simulink model "Eingangs_Ausgangs_Linearisierung_U1_2024b"  (R2024b)
settings: Solver=VariableStepAuto  StartTime=0.0  StopTime=10  MaxStep=1e-3
InitFcn:
  | clear all;
  | 
  | R = 1e+3;
  | L = 100e-3;
  | C1 = 100e-9;
  | C2 = 1e-6;
  | 
  | k  = 1.380649e-23;
  | e  = 1.602176634e-19;
  | T  = 25 + 273.15;
  | UT = k*T/e;
  | IS = 10e-9;
  | 
  | U0 = 12;
  | I0 = 10e-3;
  | 
  | syms U1 U2 IL
  | x = [U1, U2, IL];
  | 
  | %Zerlegung für Linearisierung
  | f = [-IS*exp(-U2/UT)/C1 + IL/C1;
  |      IL/C2;
  |      -U1/L - U2/L - R*IL/L];
  | 
  | g = [0, 0;
  |      0, -1/C2;
  |      1/L, 0];
  | 
  | h = U1;
  | 
  | %Lie-Ableitungen
  | Lf = h;
  | Lf_h = Lf;
  | 
  | Lf_r_init = sym(zeros(10,1));
  | Lf_r_init(1) = Lf_h;
  | 
  | r = 0;
  | 
  | 
  | while true
  | 
  |     LgLf = jacobian(Lf, x) * g;
  | 
  |     if (LgLf(1) ~= 0 || LgLf(2) ~= 0)
  |         Lf = jacobian(Lf, x) * f;
  |         Lf_h = Lf;
  |         break;
  |     end
  | 
  |     Lf = jacobian(Lf, x) * f;
  |     Lf_h = Lf;
  |     Lf_r_init(r+2) = Lf_h;
  |     r = r + 1;
  | 
  | end
  | 
  | r = r + 1
  | 
  | if r == 1
  | 
  |     Lf_r = zeros(1,1);
  |     Lf_r = Lf_r_init(1);
  | 
  |     % Pol für Regelung
  |     p = -3;
  | 
  | end
  | 
  | if r == 2
  | 
  |     Lf_r = zeros(2,1);
  |     Lf_r = Lf_r_init(1:2);
  | 
  |     % Pole für Regelung
  |     p = [-2-2*i, -2+2*i];
  | 
  | end
  | 
  | phi = Lf_r
  | 
  | alpha = LgLf;
  | alpha_pinv = pinv(alpha)
  | 
  | beta = Lf_h
  | 
  | A = zeros(r);
  | for i=1:r
  |     for j=1:r
  |         if j == i+1
  |             A(i,j) = 1;
  |         end
  |     end
  | end
  | 
  | A
  | 
  | B = zeros(r,1);
  | B(r) = 1
  | 
  | C = zeros(1,r);
  | C(1) = 1
  | 
  | p
  | 
  | G = place(A, B, p)
settings Model: Creator=richa  LastModifiedBy=richa
settings ConfigComp: CovBoundaryAbsTol=1.0e-5

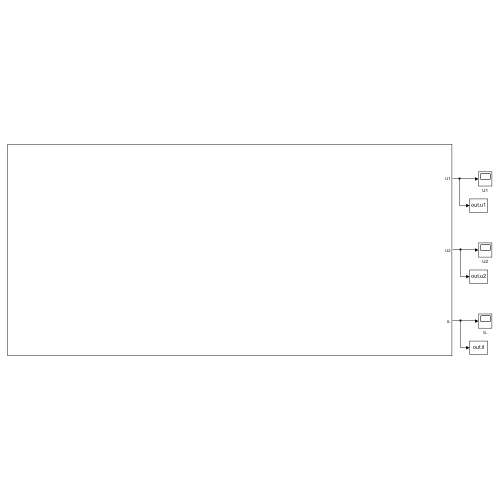
[thumbnail: Simulink's stored preview of the top-level diagram]
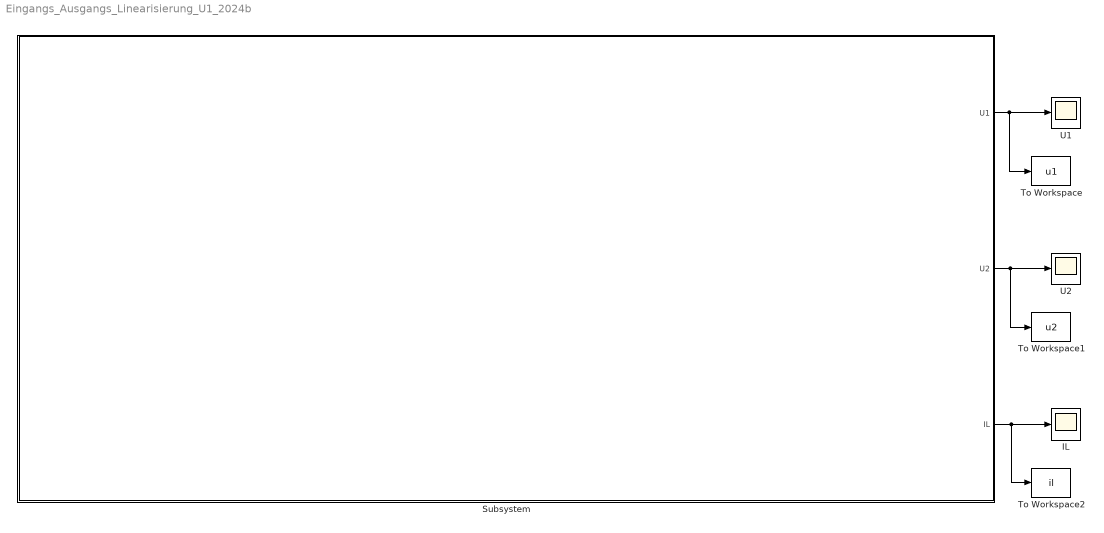
== system Eingangs_Ausgangs_Linearisierung_U1_2024b ==
  IL : Scope
  Subsystem : Subsystem
  To Workspace : ToWorkspace  VariableName=u1  SaveFormat=Structure With Time  SampleTime=-1
  To Workspace1 : ToWorkspace  VariableName=u2  SaveFormat=Structure With Time  SampleTime=-1
  To Workspace2 : ToWorkspace  VariableName=il  SaveFormat=Structure With Time  SampleTime=-1
  U1 : Scope
  U2 : Scope
  wires:
  Subsystem/1(U1) -> U1/1, To Workspace/1
  Subsystem/2(U2) -> To Workspace1/1, U2/1
  Subsystem/3(IL) -> To Workspace2/1, IL/1

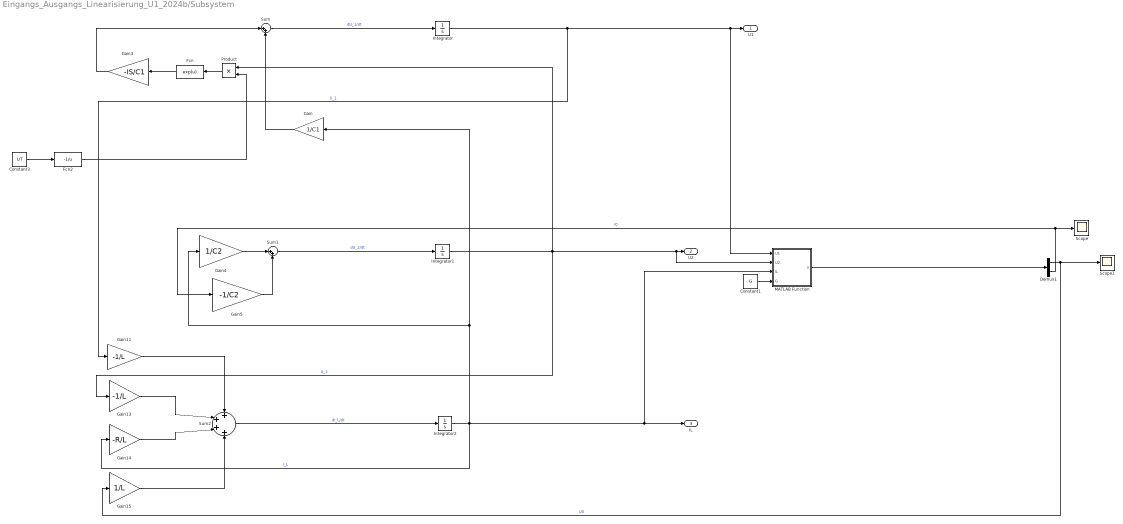
== system Eingangs_Ausgangs_Linearisierung_U1_2024b/Subsystem ==
  Constant1 : Constant  Value=G
  Constant3 : Constant  Value=UT
  Demux1 : Demux  Outputs=2
  Fcn : Fcn  Expr=exp(u)
  Fcn2 : Fcn  Expr=-1/u
  Gain : Gain  Gain=1/C1
  Gain11 : Gain  Gain=-1/L
  Gain13 : Gain  Gain=-1/L
  Gain14 : Gain  Gain=-R/L
  Gain15 : Gain  Gain=1/L
  Gain3 : Gain  Gain=-IS/C1
  Gain4 : Gain  Gain=1/C2
  Gain5 : Gain  Gain=-1/C2
  Integrator : Integrator
  Integrator1 : Integrator
  Integrator2 : Integrator
  MATLAB Function : MATLAB Function  TreatAsAtomicUnit=on
  Product : Product
  Scope : Scope
  Scope1 : Scope
  Sum : Sum  Inputs=|++
  Sum1 : Sum  Inputs=|++
  Sum2 : Sum  Inputs=++++
  U1 : Outport
  U2 : Outport  Port=2
  IL : Outport  Port=3
  wires:
  Gain4/1 -> Sum1/1
  Gain11/1 -> Sum2/1
  Fcn2/1 -> Product/2
  Gain/1 -> Sum/2
  Gain13/1 -> Sum2/2
  Gain5/1 -> Sum1/2
  Integrator1/1 -> MATLAB Function/2(U2), U2/1, Product/1, Gain13/1  "U_2"
  Gain3/1 -> Sum/1
  Sum1/1 -> Integrator1/1  "dU_2/dt"
  Integrator/1 -> MATLAB Function/1(U1), U1/1, Gain11/1  "U_1"
  Constant3/1 -> Fcn2/1
  Product/1 -> Fcn/1
  Gain14/1 -> Sum2/3
  Sum/1 -> Integrator/1  "dU_1/dt"
  Fcn/1 -> Gain3/1
  Gain15/1 -> Sum2/4
  Sum2/1 -> Integrator2/1  "dI_L/dt"
  Integrator2/1 -> MATLAB Function/3(IL), IL/1, Gain14/1, Gain/1, Gain4/1  "I_L"
  Demux1/1 -> Scope1/1, Gain15/1  "U0"
  Demux1/2 -> Scope/1, Gain5/1  "I0"
  MATLAB Function/1(u) -> Demux1/1
  Constant1/1 -> MATLAB Function/4(G)

== matlab function Eingangs_Ausgangs_Linearisierung_U1_2024b/Subsystem/MATLAB Function ==
  data: U1 input; u output; U2 input; IL input; G input
function u = fcn(U1, U2, IL, G)
    
    % z = phi(x) = phi(U1, U2, IL)
    z = [U1; 10000000*IL - exp(-(144115188075855872*U2)/3702690872189095)/10];
    
    % v = - G * (z - z_ref)
    v = -G .* (z - [10; 0]);
    
    % u = alpha^-1 * (v - beta)
    u = [100000000/((8307674973655724205648794126752153600000000*exp(-(144115188075855872*U2)/3702690872189095)*exp(-(144115188075855872*conj(U2))/3702690872189095))/548396787799697641796697476761 + 10000000000000000); -(2882303761517117440000*exp(-(144115188075855872*conj(U2))/3702690872189095))/(740538174437819*((8307674973655724205648794126752153600000000*exp(-(144115188075855872*U2)/3702690872189095)*exp(-(144115188075855872*conj(U2))/3702690872189095))/548396787799697641796697476761 + 10000000000000000))] .* (v - ((2882303761517117440000*IL*exp(-(144115188075855872*U2)/3702690872189095))/740538174437819 - 100000000*U1 - 100000000*U2 - 100000000000*IL));

end
